simulink model "flyback_PID_working(1)"  (R2022b)
settings: Solver=FixedStepDiscrete  StartTime=0.0  StopTime=100e-3  RelTol=1e-3
undefined symbols (not defined in the file): DiscIntNeverNeededParam
libraries: cstblocks x1
Description:
  | Symmetric FIR Filter
  | This example shows how to use HDL Coder(TM) to check, generate,
  | and verify HDL for a fixed-point symmetric FIR filter.
settings Model: DataTypeOverride=Off  Creator=The MathWorks, Inc.  LastModifiedBy=justu
settings SolverCC: AlgebraicLoopSolver=TrustRegion  AutoInsertRateTranBlk=on
settings DataIOCC: LimitDataPoints=on  SaveFormat=Array  SaveOutput=off  SignalLogging=off  SaveTime=off  ReturnWorkspaceOutputs=off  SignalLoggingName=logsOut
settings OptimizationCC: BlockReduction=off  BooleanDataType=off  ConditionallyExecuteInputs=off  DefaultParameterBehavior=Inlined  InheritOutputTypeSmallerThanSingle=on  InlineInvariantSignals=on  ExpressionDepthLimit=2147483647  InitFltsAndDblsToZero=on  LifeSpan=inf  BufferReusableBoundary=off
settings DebuggingCC: AlgebraicLoopMsg=error  SaveWithParameterizedLinksMsg=none  UnderspecifiedInitializationDetection=Classic  MergeDetectMultiDrivingBlocksExec=none  CheckExecutionContextPreStartOutputMsg=on  SignalResolutionControl=TryResolveAllWithWarning  MultiTaskDSMMsg=warning  MultiTaskCondExecSysMsg=none  SingleTaskRateTransMsg=error  IntegerOverflowMsg=none  ParameterPrecisionLossMsg=none  FcnCallInpInsideContextMsg=warning  UnconnectedInputMsg=warning  UnconnectedOutputMsg=warning  UnconnectedLineMsg=warning  BusObjectLabelMismatch=none  StateNameClashWarn=warning  SFUnexpectedBacktrackingDiag=warning  SFNoUnconditionalDefaultTransitionDiag=warning  SFExecutionAtInitializationDiag=none  SFMachineParentedDataDiag=warning  IntegerSaturationMsg=none  ArithmeticOperatorsInVariantConditions=warning
settings HardwareCC: ProdBitPerPointer=32  ProdBitPerSizeT=32  ProdBitPerPtrDiffT=32  ProdLargestAtomicFloat=None  ProdIntDivRoundTo=Undefined  ProdEndianess=Unspecified  ProdWordSize=32  ProdHWDeviceType=ASIC/FPGA  TargetUnknown=on  ProdEqTarget=off
settings ModelReferenceCC: EnableRefExpFcnMdlSchedulingChecks=on  PropagateSignalLabelsOutOfModel=off
settings SFSimCC: SimUseLocalCustomCode=off  CustomCodeUndefinedFunction=UseInterfaceOnly
settings RTWCC: RTWUseLocalCustomCode=off  DLArmComputeVersion=19.05
settings CodeAppCC: StateflowObjectComments=on
settings GRTTargetCC: TargetFcnLib=ansi_tfl_tmw.mat  TargetLangStandard=C89/C90 (ANSI)  CombineOutputUpdateFcns=off  GRTInterface=on
settings ConfigComp: CovMetricSettings=dw  CovSaveCumulativeToWorkspaceVar=on  CovSaveSingleToWorkspaceVar=on  CovExternalEMLEnable=off

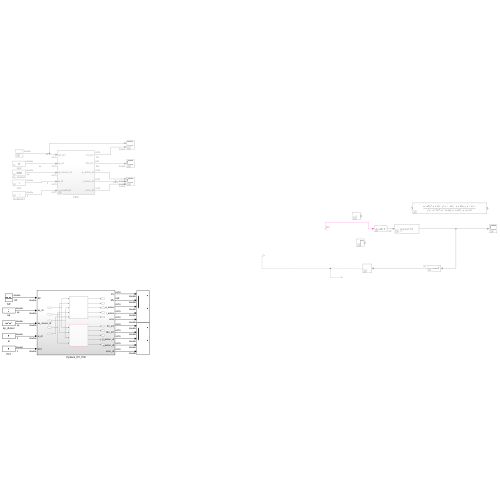
[thumbnail: Simulink's stored preview of the top-level diagram]
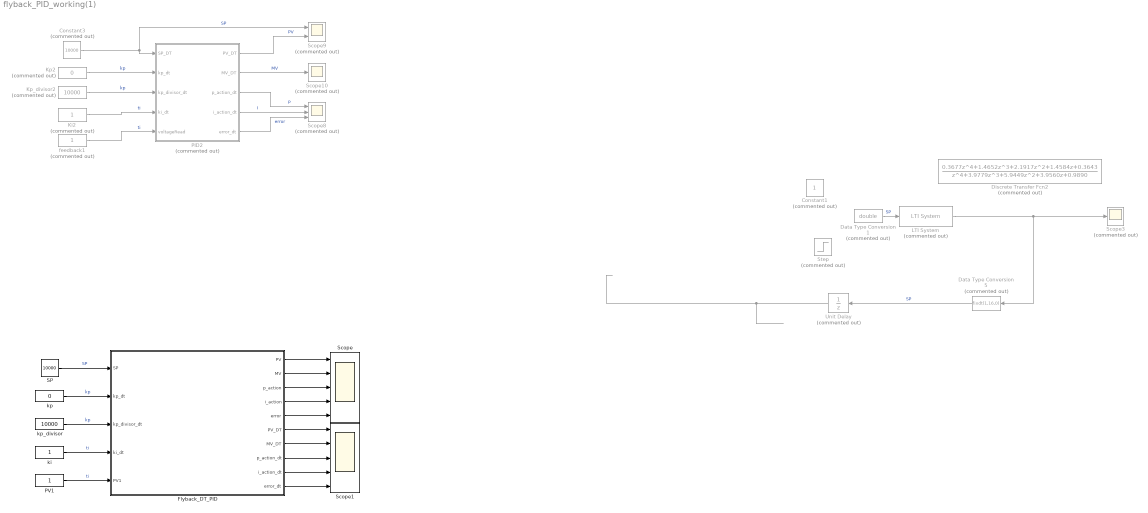
== system flyback_PID_working(1) ==
  Constant1 : Constant  Commented=on  OutDataTypeStr=fixdt(1,16,0)
  Constant3 : Constant  Commented=on  Value=10000  OutDataTypeStr=fixdt(1,16,0)
  Data Type Conversion1 : DataTypeConversion  Commented=on  OutDataTypeStr=double  SaturateOnIntegerOverflow=off  RndMeth=Floor
  Data Type Conversion5 : DataTypeConversion  Commented=on  OutDataTypeStr=fixdt(1,16,0)  SaturateOnIntegerOverflow=off  RndMeth=Floor
  Discrete Transfer Fcn2 : DiscreteTransferFcn  Commented=on  Numerator=[0.3677 1.4652 2.1917 1.4584 0.3643]  Denominator=[1 3.9779 5.9449 3.9560 0.9890]  SampleTime=0.00001  NumCoefDataTypeStr=fixdt(1,64,32)  DenCoefDataTypeStr=fixdt(1,64,32)  NumProductDataTypeStr=fixdt(1,64,32)  DenProductDataTypeStr=fixdt(1,64,32)  NumAccumDataTypeStr=fixdt(1,64,32)  DenAccumDataTypeStr=fixdt(1,64,32)  OutDataTypeStr=fixdt(1,64,32)
  Flyback_DT_PID : Subsystem
  Ki2 : Constant  Commented=on  OutDataTypeStr=fixdt(1,16,0)
  Kp2 : Constant  Commented=on  Value=0  OutDataTypeStr=fixdt(1,16,0)
  Kp_divisor2 : Constant  Commented=on  Value=10000  OutDataTypeStr=fixdt(1,16,0)
  LTI System : cstblocks/LTI System  Commented=on  sys=flybackTFD  IC=[]
  PID2 : Subsystem  Commented=on
  PV1 : Constant  OutDataTypeStr=fixdt(1,16,0)
  SP : Constant  Value=10000  OutDataTypeStr=fixdt(1,16,0)
  Scope : Scope  NumInputPorts=5
  Scope1 : Scope  NumInputPorts=5
  Scope10 : Scope  Commented=on
  Scope3 : Scope  Commented=on
  Scope8 : Scope  Commented=on  NumInputPorts=3
  Scope9 : Scope  Commented=on  NumInputPorts=2
  Step : Step  Commented=on  Time=0  After=30  SampleTime=0
  Unit Delay : UnitDelay  Commented=on  SampleTime=-1  HasFrameUpgradeWarning=on
  feedback1 : Constant  Commented=on  OutDataTypeStr=fixdt(1,16,0)
  ki : Constant  OutDataTypeStr=fixdt(1,16,0)
  kp : Constant  Value=0  OutDataTypeStr=fixdt(1,16,0)
  kp_divisor : Constant  Value=10000  OutDataTypeStr=fixdt(1,16,0)
  wires:
  Data Type Conversion1/1 -> LTI System/1  "SP"
  Data Type Conversion5/1 -> Unit Delay/1  "SP"
  Unit Delay/1 -> ?
  ? -> Data Type Conversion1/1  "MV"
  LTI System/1 -> Data Type Conversion5/1, Scope3/1
  feedback1/1 -> PID2/5(voltageRead)  "ti"
  Kp_divisor2/1 -> PID2/3(kp_divisor_dt)  "kp"
  PID2/4(i_action_dt) -> Scope8/2  "I"
  PID2/2(MV_DT) -> Scope10/1  "MV"
  PID2/1(PV_DT) -> Scope9/2  "PV"
  PID2/5(error_dt) -> Scope8/3  "error"
  PID2/3(p_action_dt) -> Scope8/1  "P"
  Constant3/1 -> Scope9/1, PID2/1(SP_DT)  "SP"
  Ki2/1 -> PID2/4(ki_dt)  "ti"
  Kp2/1 -> PID2/2(kp_dt)  "kp"
  SP/1 -> Flyback_DT_PID/1(SP)  "SP"
  kp/1 -> Flyback_DT_PID/2(kp_dt)  "kp"
  kp_divisor/1 -> Flyback_DT_PID/3(kp_divisor_dt)  "kp"
  ki/1 -> Flyback_DT_PID/4(ki_dt)  "ti"
  PV1/1 -> Flyback_DT_PID/5(PV1)  "ti"
  Flyback_DT_PID/1(PV) -> Scope/1
  Flyback_DT_PID/2(MV) -> Scope/2
  Flyback_DT_PID/3(p_action) -> Scope/3
  Flyback_DT_PID/4(i_action) -> Scope/4
  Flyback_DT_PID/5(error) -> Scope/5
  Flyback_DT_PID/6(PV_DT) -> Scope1/1
  Flyback_DT_PID/7(MV_DT) -> Scope1/2
  Flyback_DT_PID/8(p_action_dt) -> Scope1/3
  Flyback_DT_PID/9(i_action_dt) -> Scope1/4
  Flyback_DT_PID/10(error_dt) -> Scope1/5

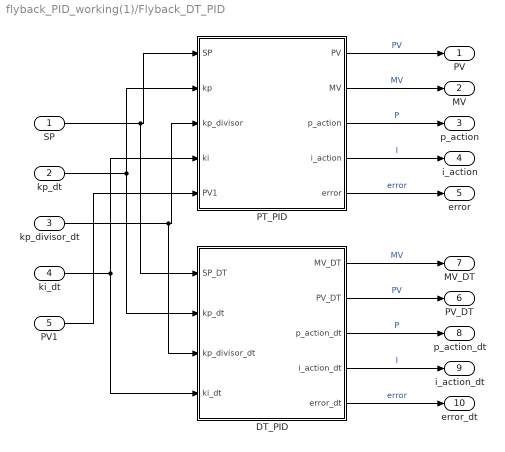
== system flyback_PID_working(1)/Flyback_DT_PID ==
  SP : Inport
  kp_dt : Inport  Port=2
  kp_divisor_dt : Inport  Port=3
  ki_dt : Inport  Port=4
  PV1 : Inport  Port=5
  DT_PID : Subsystem
  PT_PID : Subsystem
  PV : Outport  OutDataTypeStr=fixdt(1,16,0)  SampleTime=0.00001  VectorParamsAs1DForOutWhenUnconnected=off
  MV : Outport  Port=2  OutDataTypeStr=fixdt(1,8,0)  SampleTime=0.00001  VectorParamsAs1DForOutWhenUnconnected=off
  p_action : Outport  Port=3  OutDataTypeStr=fixdt(1,16,0)  SampleTime=0.00001  VectorParamsAs1DForOutWhenUnconnected=off
  i_action : Outport  Port=4  OutDataTypeStr=fixdt(1,16,0)  SampleTime=0.00001  VectorParamsAs1DForOutWhenUnconnected=off
  error : Outport  Port=5  OutDataTypeStr=fixdt(1,16,0)  SampleTime=0.00001  VectorParamsAs1DForOutWhenUnconnected=off
  PV_DT : Outport  Port=6  OutDataTypeStr=fixdt(1,16,0)  SampleTime=0.00001  VectorParamsAs1DForOutWhenUnconnected=off
  MV_DT : Outport  Port=7  OutDataTypeStr=fixdt(1,16,0)  SampleTime=0.00001  VectorParamsAs1DForOutWhenUnconnected=off
  p_action_dt : Outport  Port=8  OutDataTypeStr=fixdt(1,16,0)  SampleTime=0.00001  VectorParamsAs1DForOutWhenUnconnected=off
  i_action_dt : Outport  Port=9  OutDataTypeStr=fixdt(1,16,0)  SampleTime=0.00001  VectorParamsAs1DForOutWhenUnconnected=off
  error_dt : Outport  Port=10  OutDataTypeStr=fixdt(1,16,0)  SampleTime=0.00001  VectorParamsAs1DForOutWhenUnconnected=off
  wires:
  PT_PID/1(PV) -> PV/1  "PV"
  PT_PID/2(MV) -> MV/1  "MV"
  PT_PID/3(p_action) -> p_action/1  "P"
  PT_PID/4(i_action) -> i_action/1  "I"
  PT_PID/5(error) -> error/1  "error"
  DT_PID/1(MV_DT) -> MV_DT/1  "MV"
  DT_PID/2(PV_DT) -> PV_DT/1  "PV"
  DT_PID/3(p_action_dt) -> p_action_dt/1  "P"
  DT_PID/4(i_action_dt) -> i_action_dt/1  "I"
  DT_PID/5(error_dt) -> error_dt/1  "error"
  SP/1 -> DT_PID/1(SP_DT), PT_PID/1(SP)
  kp_dt/1 -> PT_PID/2(kp), DT_PID/2(kp_dt)
  kp_divisor_dt/1 -> DT_PID/3(kp_divisor_dt), PT_PID/3(kp_divisor)
  ki_dt/1 -> DT_PID/4(ki_dt), PT_PID/4(ki)
  PV1/1 -> PT_PID/5(PV1)

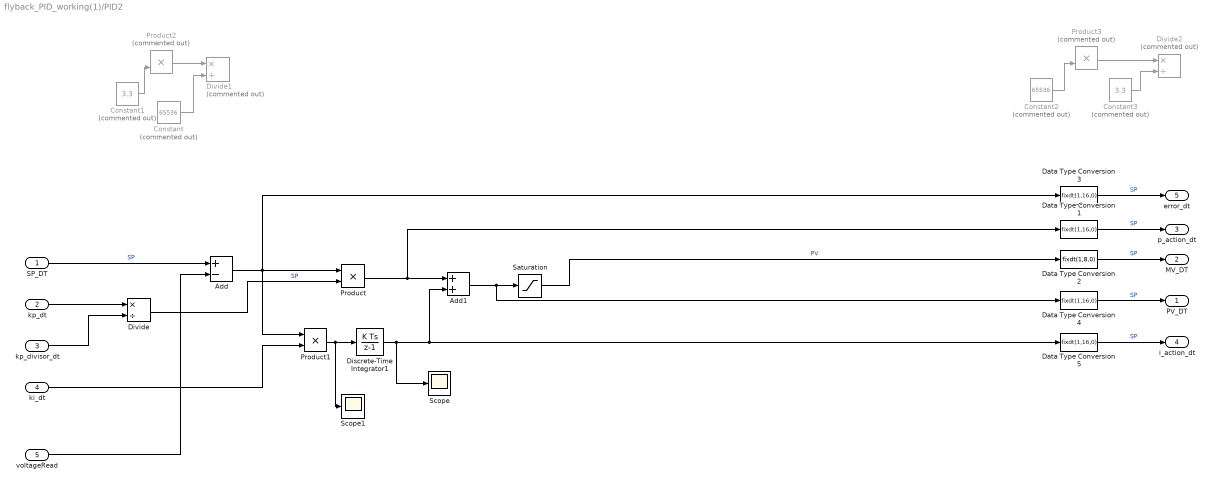
== system flyback_PID_working(1)/PID2 ==
  SP_DT : Inport  OutDataTypeStr=fixdt(1,16,0)  SampleTime=0.00001
  kp_dt : Inport  Port=2  OutDataTypeStr=fixdt(1,16,0)  SampleTime=0.00001
  kp_divisor_dt : Inport  Port=3  OutDataTypeStr=fixdt(1,16,0)  SampleTime=0.00001
  ki_dt : Inport  Port=4  OutDataTypeStr=fixdt(1,16,0)  SampleTime=0.00001
  voltageRead : Inport  Port=5  OutDataTypeStr=fixdt(1,16,0)
  Add : Sum  Inputs=+-  AccumDataTypeStr=fixdt(1,64,32)  OutDataTypeStr=fixdt(1,64,32)
  Add1 : Sum  AccumDataTypeStr=fixdt(1,64,32)  OutDataTypeStr=fixdt(1,64,32)
  Constant : Constant  Commented=on  Value=65536  OutDataTypeStr=fixdt(1,64,32)
  Constant1 : Constant  Commented=on  Value=3.3  OutDataTypeStr=fixdt(1,64,32)
  Constant2 : Constant  Commented=on  Value=65536  OutDataTypeStr=fixdt(1,64,32)
  Constant3 : Constant  Commented=on  Value=3.3  OutDataTypeStr=fixdt(1,64,32)
  Data Type Conversion{1,3..5} (4 alike) : DataTypeConversion  OutDataTypeStr=fixdt(1,16,0)  SaturateOnIntegerOverflow=off  RndMeth=Floor
  Data Type Conversion2 : DataTypeConversion  OutDataTypeStr=fixdt(1,8,0)  SaturateOnIntegerOverflow=off  RndMeth=Floor
  Discrete-Time Integrator1 : DiscreteIntegrator  SampleTime=0.00001  OutDataTypeStr=fixdt(1,64,32)  ICPrevOutput=DiscIntNeverNeededParam  ICPrevScaledInput=DiscIntNeverNeededParam
  Divide : Product  Inputs=*/  RndMeth=Zero  SaturateOnIntegerOverflow=on  LockScale=on
  Divide1 : Product  Commented=on  Inputs=*/  RndMeth=Zero  SaturateOnIntegerOverflow=on  LockScale=on
  Divide2 : Product  Commented=on  Inputs=*/  RndMeth=Zero  SaturateOnIntegerOverflow=on  LockScale=on
  Product : Product  OutDataTypeStr=fixdt(1,64,32)
  Product1 : Product  OutDataTypeStr=fixdt(1,64,32)
  Product2 : Product  Commented=on  OutDataTypeStr=fixdt(1,64,32)
  Product3 : Product  Commented=on  OutDataTypeStr=fixdt(1,64,32)
  Saturation : Saturate  UpperLimit=255  LowerLimit=0  OutDataTypeStr=fixdt(1,64,32)
  Scope : Scope
  Scope1 : Scope
  PV_DT : Outport  OutDataTypeStr=fixdt(1,16,0)  SampleTime=0.00001  VectorParamsAs1DForOutWhenUnconnected=off
  MV_DT : Outport  Port=2  OutDataTypeStr=fixdt(1,8,0)  SampleTime=0.00001  VectorParamsAs1DForOutWhenUnconnected=off
  p_action_dt : Outport  Port=3  OutDataTypeStr=fixdt(1,16,0)  SampleTime=0.00001  VectorParamsAs1DForOutWhenUnconnected=off
  i_action_dt : Outport  Port=4  OutDataTypeStr=fixdt(1,16,0)  SampleTime=0.00001  VectorParamsAs1DForOutWhenUnconnected=off
  error_dt : Outport  Port=5  OutDataTypeStr=fixdt(1,16,0)  SampleTime=0.00001  VectorParamsAs1DForOutWhenUnconnected=off
  wires:
  voltageRead/1 -> Add/2
  Product3/1 -> Divide2/1
  Constant2/1 -> Product3/2
  Constant3/1 -> Divide2/2
  Constant/1 -> Divide1/2
  Constant1/1 -> Product2/2
  Product2/1 -> Divide1/1
  SP_DT/1 -> Add/1  "SP"
  Add1/1 -> Saturation/1, Data Type Conversion4/1
  Divide/1 -> Product/2  "SP"
  kp_divisor_dt/1 -> Divide/2
  kp_dt/1 -> Divide/1
  ki_dt/1 -> Product1/2
  Data Type Conversion5/1 -> i_action_dt/1  "SP"
  Data Type Conversion4/1 -> PV_DT/1  "SP"
  Data Type Conversion2/1 -> MV_DT/1  "SP"
  Data Type Conversion3/1 -> error_dt/1  "SP"
  Data Type Conversion1/1 -> p_action_dt/1  "SP"
  Discrete-Time Integrator1/1 -> Add1/2, Data Type Conversion5/1, Scope/1
  Saturation/1 -> Data Type Conversion2/1  "PV"
  Product/1 -> Add1/1, Data Type Conversion1/1
  Add/1 -> Product1/1, Product/1, Data Type Conversion3/1
  Product1/1 -> Discrete-Time Integrator1/1, Scope1/1

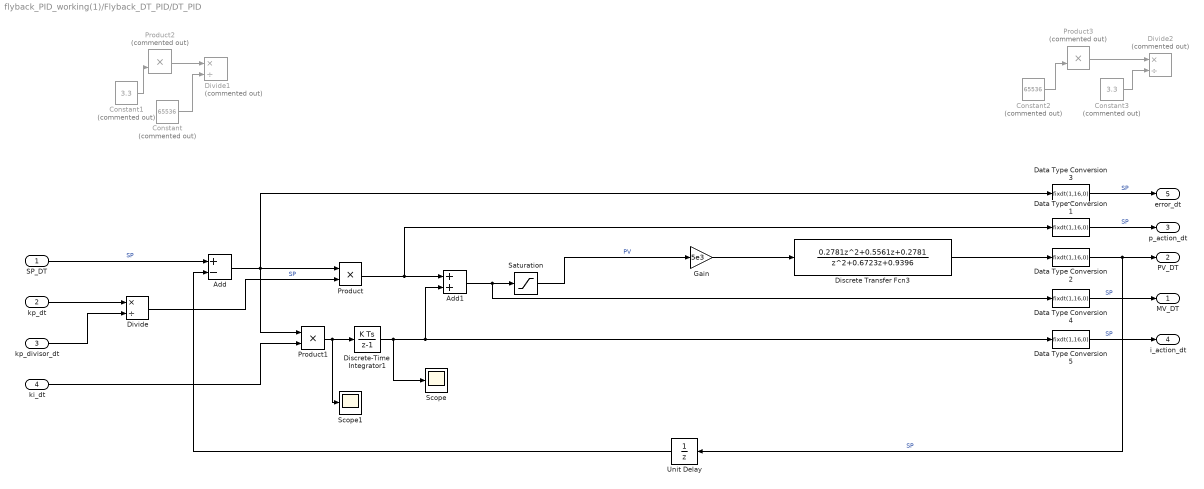
== system flyback_PID_working(1)/Flyback_DT_PID/DT_PID ==
  SP_DT : Inport  OutDataTypeStr=fixdt(1,16,0)  SampleTime=0.00001
  kp_dt : Inport  Port=2  OutDataTypeStr=fixdt(1,16,0)  SampleTime=0.00001
  kp_divisor_dt : Inport  Port=3  OutDataTypeStr=fixdt(1,16,0)  SampleTime=0.00001
  ki_dt : Inport  Port=4  OutDataTypeStr=fixdt(1,16,0)  SampleTime=0.00001
  Add : Sum  Inputs=+-  AccumDataTypeStr=fixdt(1,64,32)  OutDataTypeStr=fixdt(1,64,32)
  Add1 : Sum  AccumDataTypeStr=fixdt(1,64,32)  OutDataTypeStr=fixdt(1,64,32)
  Constant : Constant  Commented=on  Value=65536  OutDataTypeStr=fixdt(1,64,32)
  Constant1 : Constant  Commented=on  Value=3.3  OutDataTypeStr=fixdt(1,64,32)
  Constant2 : Constant  Commented=on  Value=65536  OutDataTypeStr=fixdt(1,64,32)
  Constant3 : Constant  Commented=on  Value=3.3  OutDataTypeStr=fixdt(1,64,32)
  Data Type Conversion{1..5} (5 alike) : DataTypeConversion  OutDataTypeStr=fixdt(1,16,0)  SaturateOnIntegerOverflow=off  RndMeth=Floor
  Discrete Transfer Fcn3 : DiscreteTransferFcn  Numerator=[0.2781 0.5561 0.2781]  Denominator=[1 0.6723 0.9396]  SampleTime=1e-5  a0EqualsOne=on  NumCoefDataTypeStr=fixdt(1,64,32)  DenCoefDataTypeStr=fixdt(1,64,32)  NumProductDataTypeStr=fixdt(1,64,32)  DenProductDataTypeStr=fixdt(1,64,32)  NumAccumDataTypeStr=fixdt(1,64,32)  DenAccumDataTypeStr=fixdt(1,64,32)  OutDataTypeStr=fixdt(1,64,32)
  Discrete-Time Integrator1 : DiscreteIntegrator  SampleTime=0.00001  OutDataTypeStr=fixdt(1,64,32)  ICPrevOutput=DiscIntNeverNeededParam  ICPrevScaledInput=DiscIntNeverNeededParam
  Divide : Product  Inputs=*/  RndMeth=Zero  SaturateOnIntegerOverflow=on  LockScale=on
  Divide1 : Product  Commented=on  Inputs=*/  RndMeth=Zero  SaturateOnIntegerOverflow=on  LockScale=on
  Divide2 : Product  Commented=on  Inputs=*/  RndMeth=Zero  SaturateOnIntegerOverflow=on  LockScale=on
  Gain : Gain  Gain=5e3
  Product : Product  OutDataTypeStr=fixdt(1,64,32)
  Product1 : Product  OutDataTypeStr=fixdt(1,64,32)
  Product2 : Product  Commented=on  OutDataTypeStr=fixdt(1,64,32)
  Product3 : Product  Commented=on  OutDataTypeStr=fixdt(1,64,32)
  Saturation : Saturate  UpperLimit=255  LowerLimit=0  OutDataTypeStr=fixdt(1,64,32)
  Scope : Scope
  Scope1 : Scope
  Unit Delay : UnitDelay  SampleTime=-1  HasFrameUpgradeWarning=on
  MV_DT : Outport  OutDataTypeStr=fixdt(1,16,0)  SampleTime=0.00001  VectorParamsAs1DForOutWhenUnconnected=off
  PV_DT : Outport  Port=2  OutDataTypeStr=fixdt(1,16,0)  SampleTime=0.00001  VectorParamsAs1DForOutWhenUnconnected=off
  p_action_dt : Outport  Port=3  OutDataTypeStr=fixdt(1,16,0)  SampleTime=0.00001  VectorParamsAs1DForOutWhenUnconnected=off
  i_action_dt : Outport  Port=4  OutDataTypeStr=fixdt(1,16,0)  SampleTime=0.00001  VectorParamsAs1DForOutWhenUnconnected=off
  error_dt : Outport  Port=5  OutDataTypeStr=fixdt(1,16,0)  SampleTime=0.00001  VectorParamsAs1DForOutWhenUnconnected=off
  wires:
  Product3/1 -> Divide2/1
  Constant2/1 -> Product3/2
  Constant3/1 -> Divide2/2
  Constant/1 -> Divide1/2
  Constant1/1 -> Product2/2
  Product2/1 -> Divide1/1
  SP_DT/1 -> Add/1  "SP"
  Add1/1 -> Saturation/1, Data Type Conversion4/1
  Divide/1 -> Product/2  "SP"
  kp_divisor_dt/1 -> Divide/2
  kp_dt/1 -> Divide/1
  ki_dt/1 -> Product1/2
  Data Type Conversion5/1 -> i_action_dt/1  "SP"
  Data Type Conversion4/1 -> MV_DT/1  "SP"
  Data Type Conversion2/1 -> Unit Delay/1, PV_DT/1  "SP"
  Data Type Conversion3/1 -> error_dt/1  "SP"
  Data Type Conversion1/1 -> p_action_dt/1  "SP"
  Discrete-Time Integrator1/1 -> Add1/2, Data Type Conversion5/1, Scope/1
  Saturation/1 -> Gain/1  "PV"
  Product/1 -> Add1/1, Data Type Conversion1/1
  Add/1 -> Product1/1, Product/1, Data Type Conversion3/1
  Product1/1 -> Discrete-Time Integrator1/1, Scope1/1
  Discrete Transfer Fcn3/1 -> Data Type Conversion2/1
  Unit Delay/1 -> Add/2
  Gain/1 -> Discrete Transfer Fcn3/1

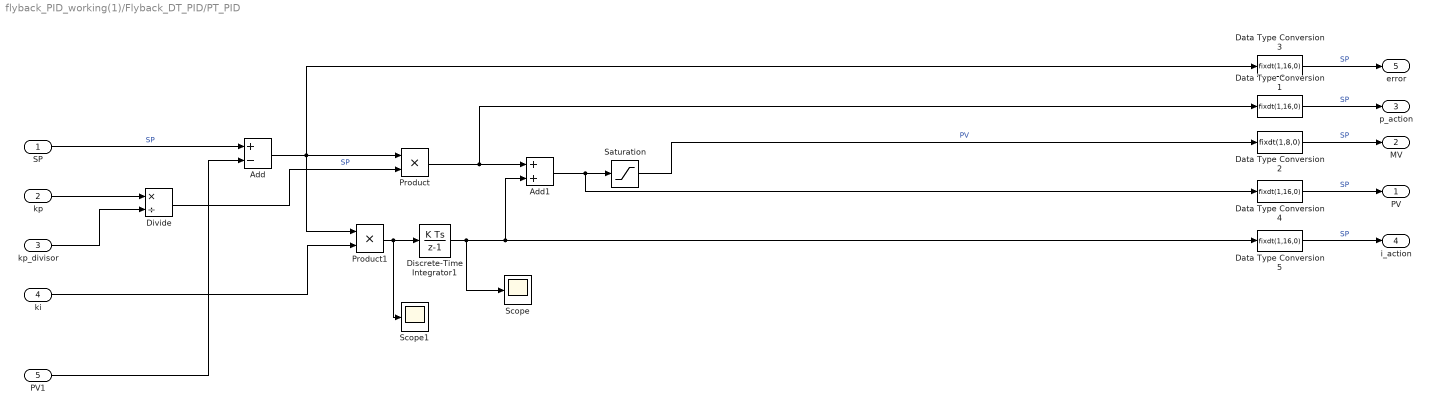
== system flyback_PID_working(1)/Flyback_DT_PID/PT_PID ==
  SP : Inport  OutDataTypeStr=fixdt(1,16,0)  SampleTime=0.00001
  kp : Inport  Port=2  OutDataTypeStr=fixdt(1,16,0)  SampleTime=0.00001
  kp_divisor : Inport  Port=3  OutDataTypeStr=fixdt(1,16,0)  SampleTime=0.00001
  ki : Inport  Port=4  OutDataTypeStr=fixdt(1,16,0)  SampleTime=0.00001
  PV1 : Inport  Port=5  OutDataTypeStr=fixdt(1,16,0)
  Add : Sum  Inputs=+-  AccumDataTypeStr=fixdt(1,64,32)  OutDataTypeStr=fixdt(1,64,32)
  Add1 : Sum  AccumDataTypeStr=fixdt(1,64,32)  OutDataTypeStr=fixdt(1,64,32)
  Data Type Conversion{1,3..5} (4 alike) : DataTypeConversion  OutDataTypeStr=fixdt(1,16,0)  SaturateOnIntegerOverflow=off  RndMeth=Floor
  Data Type Conversion2 : DataTypeConversion  OutDataTypeStr=fixdt(1,8,0)  SaturateOnIntegerOverflow=off  RndMeth=Floor
  Discrete-Time Integrator1 : DiscreteIntegrator  SampleTime=0.00001  OutDataTypeStr=fixdt(1,64,32)  ICPrevOutput=DiscIntNeverNeededParam  ICPrevScaledInput=DiscIntNeverNeededParam
  Divide : Product  Inputs=*/  RndMeth=Zero  SaturateOnIntegerOverflow=on  LockScale=on
  Product : Product  OutDataTypeStr=fixdt(1,64,32)
  Product1 : Product  OutDataTypeStr=fixdt(1,64,32)
  Saturation : Saturate  UpperLimit=255  LowerLimit=0  OutDataTypeStr=fixdt(1,64,32)
  Scope : Scope
  Scope1 : Scope
  PV : Outport  OutDataTypeStr=fixdt(1,16,0)  SampleTime=0.00001  VectorParamsAs1DForOutWhenUnconnected=off
  MV : Outport  Port=2  OutDataTypeStr=fixdt(1,8,0)  SampleTime=0.00001  VectorParamsAs1DForOutWhenUnconnected=off
  p_action : Outport  Port=3  OutDataTypeStr=fixdt(1,16,0)  SampleTime=0.00001  VectorParamsAs1DForOutWhenUnconnected=off
  i_action : Outport  Port=4  OutDataTypeStr=fixdt(1,16,0)  SampleTime=0.00001  VectorParamsAs1DForOutWhenUnconnected=off
  error : Outport  Port=5  OutDataTypeStr=fixdt(1,16,0)  SampleTime=0.00001  VectorParamsAs1DForOutWhenUnconnected=off
  wires:
  Product1/1 -> Scope1/1, Discrete-Time Integrator1/1
  Add/1 -> Data Type Conversion3/1, Product/1, Product1/1
  Product/1 -> Data Type Conversion1/1, Add1/1
  Saturation/1 -> Data Type Conversion2/1  "PV"
  Discrete-Time Integrator1/1 -> Scope/1, Data Type Conversion5/1, Add1/2
  Data Type Conversion1/1 -> p_action/1  "SP"
  Data Type Conversion3/1 -> error/1  "SP"
  Data Type Conversion2/1 -> MV/1  "SP"
  Data Type Conversion4/1 -> PV/1  "SP"
  Data Type Conversion5/1 -> i_action/1  "SP"
  ki/1 -> Product1/2
  kp/1 -> Divide/1
  kp_divisor/1 -> Divide/2
  Divide/1 -> Product/2  "SP"
  Add1/1 -> Data Type Conversion4/1, Saturation/1
  SP/1 -> Add/1  "SP"
  PV1/1 -> Add/2
